simulink model "ssc_car_fuel_cell_1motor"  (R2026a)
settings: Solver=daessc  StopTime=195  FixedStep=1e-3  AbsTol=1e-3
InitFcn:
  | %Vehicle = sm_car_vehcfg_checkConfig(Vehicle);
undefined symbols (not defined in the file): Control, Driver, Init, Maneuver1, Vehicle
libraries: fl_lib x93, nesl_utility x38, GasN_lib x21, sdl_lib x10, simulink_extras x6, SimscapeFluids_lib x6, simulink x5, customMath_lib x5, slpidlib x4, ee_lib x3, autolibshared x2, sl_discontinuities x2
(part 3 of 4)

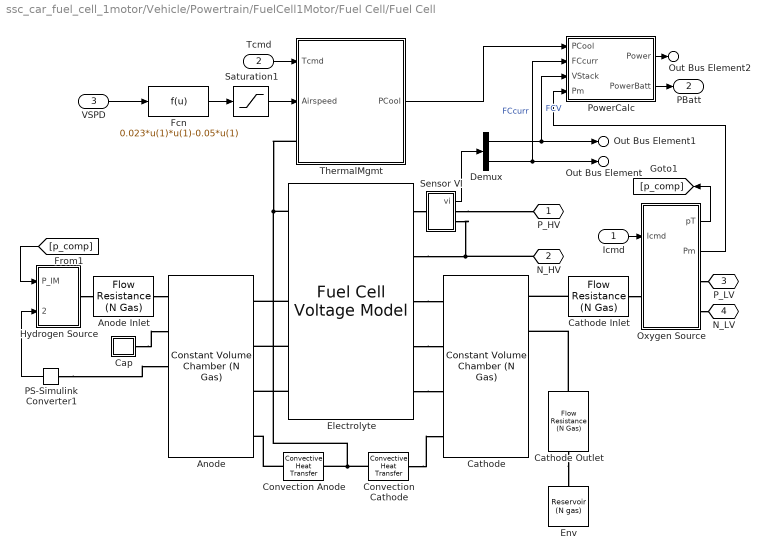
== system ssc_car_fuel_cell_1motor/Vehicle/Powertrain/FuelCell1Motor/Fuel Cell/Fuel Cell ==
  Icmd : Inport
  Tcmd : Inport  Port=2
  VSPD : Inport  Port=3
  Anode : GasN_lib/Constant Volume Chamber (N Gas)  V0=FuelCell.Anode.volume.Value m^3  p0=FuelCell.Anode.p.Value MPa  T0=FuelCell.Anode.T.Value degC  comp=GasN.composition_enum.mole  y0=FuelCell.Anode.rMoleFractions.Value'  x0=[1; 0; 0; 0]  tau_c=FuelCell.Anode.timeCondensation.Value s  is_cond=FuelCell.Anode.speciesCondensed.Value'  out_comp=GasN.composition_enum.mass  area_A=FuelCell.Anode.areaPort.Value cm^2  area_B=FuelCell.Anode.areaPort.Value cm^2  area_C=FuelCell.Anode.areaPort.Value cm^2
  Anode Inlet : GasN_lib/Flow Resistance (N Gas)  var_res=false  delta_p_nominal="FuelCell.AnodeInlet.pDropNominal.Value  MPa"  mdot_nominal=FuelCell.AnodeInlet.mdotNominal.Value kg/s  rho_nominal="FuelCell.AnodeInlet.rhoNominal.Value  kg/m^3"  laminar_fraction=FuelCell.AnodeInlet.rmdotLaminar.Value  area=FuelCell.AnodeInlet.areaPort.Value cm^2  leak_thresh=FuelCell.AnodeInlet.leakageThreshold.Value
  Cap : Subsystem
  Cathode : GasN_lib/Constant Volume Chamber (N Gas)  V0=FuelCell.Cathode.volume.Value m^3  p0=FuelCell.Cathode.p.Value MPa  T0=FuelCell.Cathode.T.Value degC  comp=GasN.composition_enum.mole  y0=FuelCell.Cathode.rMoleFractions.Value'  x0=[1; 0; 0; 0]  tau_c=FuelCell.Cathode.timeCondensation.Value s  is_cond=FuelCell.Cathode.speciesCondensed.Value'  out_comp=GasN.composition_enum.mass  area_A=FuelCell.Cathode.areaPort.Value cm^2  area_B=FuelCell.Cathode.areaPort.Value cm^2  area_C=FuelCell.Cathode.areaPort.Value cm^2
  Cathode Inlet : GasN_lib/Flow Resistance (N Gas)  var_res=false  delta_p_nominal=FuelCell.CathodeInlet.pDropNominal.Value MPa  mdot_nominal=FuelCell.CathodeInlet.mdotNominal.Value kg/s  rho_nominal="FuelCell.CathodeInlet.rhoNominal.Value  kg/m^3"  laminar_fraction=FuelCell.CathodeInlet.rmdotLaminar.Value  area=FuelCell.CathodeInlet.areaPort.Value cm^2  leak_thresh=FuelCell.CathodeInlet.leakageThreshold.Value
  Cathode Outlet : GasN_lib/Flow Resistance (N Gas)  var_res=false  delta_p_nominal=FuelCell.CathodeOutlet.pDropNominal.Value MPa  mdot_nominal=FuelCell.CathodeOutlet.mdotNominal.Value kg/s  rho_nominal=FuelCell.CathodeOutlet.rhoNominal.Value kg/m^3  laminar_fraction=FuelCell.CathodeOutlet.rmdotLaminar.Value  area=FuelCell.CathodeOutlet.areaPort.Value cm^2  leak_thresh=FuelCell.CathodeOutlet.leakageThreshold.Value
  Convection Anode : fl_lib/Thermal/Thermal Elements/Convective Heat Transfer  thermal_type=foundation.enum.constant_variable.constant  area=280*400/8 cm^2  heat_tr_coeff=10 W/(m^2 * K)  min_heat_tr_coeff=1e-3 W/(K*m^2)  T_specify=off  T_priority=None  T=0 K  T_nominal_specify=off  T_nominal_value=1  T_nominal_unit=K  Q_specify=off  Q_priority=None  Q=0 W  Q_nominal_specify=off  Q_nominal_value=1  Q_nominal_unit=W
  Convection Cathode : fl_lib/Thermal/Thermal Elements/Convective Heat Transfer  thermal_type=foundation.enum.constant_variable.constant  area=280*400/8 cm^2  heat_tr_coeff=10 W/(m^2 * K)  min_heat_tr_coeff=1e-3 W/(K*m^2)  T_specify=off  T_priority=None  T=0 K  T_nominal_specify=off  T_nominal_value=1  T_nominal_unit=K  Q_specify=off  Q_priority=None  Q=0 W  Q_nominal_specify=off  Q_nominal_value=1  Q_nominal_unit=W
  Demux : Demux  Outputs=2
  Electrolyte : gn_supplement_lib/fuel_cell/Fuel Cell Voltage Model  Ncell=FuelCell.Electrolyte.numCells.Value  Acell=FuelCell.Electrolyte.areaCell.Value cm^2  tcell=FuelCell.Electrolyte.thicknessMembrane.Value cm  io=FuelCell.Electrolyte.exchangeCurrentDensity.Value A/cm^2  iL=FuelCell.Electrolyte.maxCurrentDensity.Value A/cm^2  alpha=FuelCell.Electrolyte.transferCoefficientB.Value  rho_m=FuelCell.Electrolyte.rhoMembrane.Value kg/cm^3  M_m=FuelCell.Electrolyte.mMembrane.Value kg/mol
  Env : GasN_lib/Reservoir (N gas)  p0=FuelCell.CathodeReservoir.p.Value MPa  T0=FuelCell.CathodeReservoir.T.Value degC  constCond=true  comp=GasN.composition_enum.mole  y0=FuelCell.CathodeReservoir.rMoleFractions.Value'  x0=[1; 0; 0; 0]  area=FuelCell.CathodeReservoir.areaPort.Value cm^2
  Fcn : Fcn  Expr=0.023*u(1)*u(1)-0.05*u(1)
  Hydrogen Source : Subsystem
  Oxygen Source : Subsystem
  PS-Simulink Converter1 : nesl_utility/PS-Simulink Converter  PhysicalDomain=network_engine_domain  SubClassName=ps_output  LeftPortType=input  RightPortType=output  PseudoPeriodic=off  Frequencies=[]  VectorFormat=1-D array  Unit=Pa  AffineConversion=off
  PowerCalc : Subsystem
  Saturation1 : Saturate  UpperLimit=inf  LowerLimit=0  ZeroCross=off
  Sensor VI : Subsystem
  ThermalMgmt : Subsystem
      mask Display: image('sm_car_vehicle_power_cooling_active1loop_IMAGE.png');
  P_HV : PMIOPort  Side=Right
  N_HV : PMIOPort  Port=2  Side=Right
  P_LV : PMIOPort  Port=3  Side=Right
  N_LV : PMIOPort  Port=4  Side=Right
  Out Bus Element : Outport  PortName=m  Element=i
  Out Bus Element1 : Outport  PortName=m  Element=v
  Out Bus Element2 : Outport  PortName=m  Element=Power
  PBatt : Outport  Port=2
  wires:
  Icmd/1 -> Oxygen Source/1(Icmd)
  [p_comp] -> Hydrogen Source/1(P_IM)
  PowerCalc/1(Power) -> Out Bus Element2/1
  VSPD/1 -> Fcn/1
  Demux/2 -> PowerCalc/2(FCcurr), Out Bus Element/1  "FCcurr"
  Sensor VI/1(vi) -> Demux/1
  Fcn/1 -> Saturation1/1
  PowerCalc/2(PowerBatt) -> PBatt/1
  Tcmd/1 -> ThermalMgmt/1(Tcmd)
  Demux/1 -> PowerCalc/3(VStack), Out Bus Element1/1  "FCV"
  Oxygen Source/2(Pm) -> PowerCalc/4(Pm)
  Oxygen Source/1(pT) -> [p_comp]
  PS-Simulink Converter1/1 -> Hydrogen Source/2(P_anode)
  Saturation1/1 -> ThermalMgmt/2(Airspeed)
  ThermalMgmt/1(PCool) -> PowerCalc/1(PCool)
  connections:
  Cap/LConn1 -- Anode/RConn2
  Convection Anode/LConn1 -- Anode/LConn4
  Convection Cathode/LConn1 -- Cathode/LConn4
  Electrolyte/RConn3 -- Cathode/LConn1
  Electrolyte/RConn1 -- Sensor VI/LConn1
  Sensor VI/RConn1 -- P_HV/RConn1
  Cathode Inlet/RConn1 -- Cathode/RConn1
  Anode Inlet/RConn1 -- Anode/RConn1
  Electrolyte/LConn4 -- Anode/LConn2
  Electrolyte/RConn4 -- Cathode/LConn2
  PS-Simulink Converter1/LConn1 -- Anode/RConn3
  Oxygen Source/RConn2 -- N_LV/RConn1
  Hydrogen Source/RConn1 -- Anode Inlet/LConn1
  Electrolyte/RConn5 -- Cathode/LConn3
  Electrolyte/LConn5 -- Anode/LConn3
  Cathode Outlet/RConn1 -- Env/LConn1
  Cathode Inlet/LConn1 -- Oxygen Source/LConn1
  Oxygen Source/RConn1 -- P_LV/RConn1
  Electrolyte/LConn3 -- Anode/LConn1
  Cathode Outlet/LConn1 -- Cathode/RConn2
  Convection Anode/RConn1 -- Convection Cathode/RConn1 -- Electrolyte/LConn1 -- ThermalMgmt/LConn1
  Sensor VI/RConn2 -- Electrolyte/RConn2 -- N_HV/RConn1

== system ssc_car_fuel_cell_1motor/Vehicle/Powertrain/FuelCell1Motor/Fuel Cell/Thermal ==
  Controlled Heat Flow Rate Source : fl_lib/Thermal/Thermal Sources/Controlled Heat Flow Rate Source
  PS Gain : fl_lib/Physical Signals/Functions/PS Gain  Commented=on  gain=FuelCell.Converter.resistance.Value Ohm
  PS Math Function : fl_lib/Physical Signals/Functions/PS Math Function  Commented=on  fcn_choice=foundation.enum.math_function.square  v=1
  PS Power Function : customMath_lib/PS Power Function  resistance=FuelCell.Converter.resistance.Value Ohm
  Thermal Mass : fl_lib/Thermal/Thermal Elements/Thermal Mass  mass_type=foundation.enum.constant_variable.constant  mass=FuelCell.Converter.mThermal.Value kg  sp_heat=FuelCell.Converter.Cp.Value J/kg/K  mass_min=1e-6 kg  num_ports=foundation.enum.numPorts2.one  m_specify=off  m_priority=High  m=1 kg  m_nominal_specify=off  m_nominal_value=1  m_nominal_unit=kg  T_specify=off  T_priority=High  T=300 K  T_nominal_specify=off  T_nominal_value=1  T_nominal_unit=K  Q_specify=off  Q_priority=None  Q=0 W  Q_nominal_specify=off  Q_nominal_value=1  Q_nominal_unit=W
  Thermal Resistance : fl_lib/Thermal/Thermal Elements/Thermal Resistance  resistance=FuelCell.Converter.rConvection.Value K/W  T_specify=off  T_priority=None  T=0 K  T_nominal_specify=off  T_nominal_value=1  T_nominal_unit=K  Q_specify=off  Q_priority=None  Q=0 W  Q_nominal_specify=off  Q_nominal_value=1  Q_nominal_unit=W
  Thermal Reference2 : fl_lib/Thermal/Thermal Elements/Thermal Reference
  H : PMIOPort  Side=Right
  i : PMIOPort  Port=2  Side=Left
  connections:
  H/RConn1 -- Thermal Resistance/RConn1
  PS Power Function/LConn1 -- i/RConn1
  Thermal Reference2/LConn1 -- Controlled Heat Flow Rate Source/RConn2
  Controlled Heat Flow Rate Source/LConn1 -- Thermal Mass/LConn1 -- Thermal Resistance/LConn1
  PS Math Function/RConn1 -- PS Gain/LConn1
  PS Power Function/RConn1 -- Controlled Heat Flow Rate Source/RConn1

== system ssc_car_fuel_cell_1motor/Vehicle/Powertrain/FuelCell1Motor/Motor A1/Sensing Current ==
  Current Sensor : fl_lib/Electrical/Electrical Sensors/Current Sensor
  PS-Simulink Converter : nesl_utility/PS-Simulink Converter  PhysicalDomain=network_engine_domain  SubClassName=ps_output  LeftPortType=input  RightPortType=output  PseudoPeriodic=off  Frequencies=[]  VectorFormat=1-D array  Unit=A  AffineConversion=off
  + : PMIOPort  Side=Right
  - : PMIOPort  Port=2  Side=Left
  i : Outport
  wires:
  PS-Simulink Converter/1 -> i/1
  connections:
  Current Sensor/RConn2 -- -/RConn1
  Current Sensor/LConn1 -- +/RConn1
  PS-Simulink Converter/LConn1 -- Current Sensor/RConn1

== system ssc_car_fuel_cell_1motor/Vehicle/Powertrain/FuelCell1Motor/Motor A1/Sensing Torque ==
  PS-Simulink Converter : nesl_utility/PS-Simulink Converter  PhysicalDomain=network_engine_domain  SubClassName=ps_output  LeftPortType=input  RightPortType=output  PseudoPeriodic=off  Frequencies=[]  VectorFormat=1-D array  Unit=N*m  AffineConversion=off
  Torque Sensor : fl_lib/Mechanical/Mechanical Sensors/Ideal Torque Sensor
  C : PMIOPort  Side=Right
  R : PMIOPort  Port=2  Side=Left
  trq : Outport
  wires:
  PS-Simulink Converter/1 -> trq/1
  connections:
  Torque Sensor/LConn1 -- R/RConn1
  Torque Sensor/RConn1 -- C/RConn1
  Torque Sensor/RConn2 -- PS-Simulink Converter/LConn1

== system ssc_car_fuel_cell_1motor/Vehicle/Powertrain/FuelCell1Motor/Thermal System/Pump Control ==
  TAmb : Inport
  TMotor : Inport  Port=2
  Add : Sum  Inputs=|-+
  PID Controller : slpidlib/PID Controller  Controller=PI  Form=Parallel  TimeDomain=Continuous-time  UseExternalTs=off  SampleTime=-1  IntegratorMethod=Forward Euler  FilterMethod=Forward Euler  ControllerParametersSource=internal  P=Cooling.Control.Kp.Value  I=Cooling.Control.Ki.Value  UseKiTs=off  D=0  UseExternalDerivativeSource=off  N=100  UseFilter=on  TunerSelectOption=Transfer Function Based (PID Tuner App)  ZeroCross=off  InitialConditionSource=internal  InitialConditionForIntegrator=0  InitialConditionForFilter=0  DifferentiatorICPrevScaledInput=0  ExternalReset=none  TrackingMode=off  Kt=1  LimitOutput=on  SatLimitsSource=internal  UpperSaturationLimit=0.1  LowerSaturationLimit=0  LinearizeAsGain=on  AntiWindupMode=none  Kb=1  LimitIntegrator=off  UpperIntegratorSaturationLimit=inf  LowerIntegratorSaturationLimit=-inf  POutMin=[]  POutMax=[]  IOutMin=[]  IOutMax=[]  DOutMin=[]  DOutMax=[]  NOutMin=[]  NOutMax=[]  SumOutMin=[]  SumOutMax=[]  SaturationOutMin=[]  SaturationOutMax=[]  PParamMin=[]  PParamMax=[]  IParamMin=[]  IParamMax=[]  DParamMin=[]  DParamMax=[]  NParamMin=[]  NParamMax=[]  KbParamMin=[]  KbParamMax=[]  KtParamMin=[]  KtParamMax=[]  KbOutMin=[]  KbOutMax=[]  KtOutMin=[]  KtOutMax=[]  IntegratorOutMin=[]  IntegratorOutMax=[]  FilterOutMin=[]  FilterOutMax=[]  SumI1OutMin=[]  SumI1OutMax=[]  SumI2OutMin=[]  SumI2OutMax=[]  SumI3OutMin=[]  SumI3OutMax=[]  SumI4OutMin=[]  SumI4OutMax=[]  SumDOutMin=[]  SumDOutMax=[]  DifferentiatorOutMin=[]  DifferentiatorOutMax=[]  FilterDiffOutCoefMin=[]  FilterDiffOutCoefMax=[]  ReciprocalOutMin=[]  ReciprocalOutMax=[]  SumDenOutMin=[]  SumDenOutMax=[]  SumNumOutMin=[]  SumNumOutMax=[]  DivideOutMin=[]  DivideOutMax=[]  UdiffTsProdOutMin=[]  UdiffTsProdOutMax=[]  NTsProdOutMin=[]  NTsProdOutMax=[]  UintegralTsProdOutMin=[]  UintegralTsProdOutMax=[]  UngainTsProdOutMin=[]  UngainTsProdOutMax=[]  ClampingZeroOutDataTypeStr=Inherit: Inherit via back propagation  ClampingZeroOutMin=[]  ClampingZeroOutMax=[]  FilterDenConstantOutDataTypeStr=Inherit: Inherit via back propagation  FilterDenConstantOutMin=[]  FilterDenConstantOutMax=[]  PCopyOutDataTypeStr=Inherit: Inherit via back propagation  PCopyOutMin=[]  PCopyOutMax=[]  NCopyOutDataTypeStr=Inherit: Inherit via back propagation  NCopyOutMin=[]  NCopyOutMax=[]  IntegratorContinuousStateAttributes=''  IntegratorStateMustResolveToSignalObject=off  IntegratorRTWStateStorageClass=Auto  FilterContinuousStateAttributes=''  FilterStateMustResolveToSignalObject=off  FilterRTWStateStorageClass=Auto  ParallelPVariant=InternalParameters  IdealPVariant=Disabled  IVariant=InternalParameters  DVariant=Disabled  IntegratorVariant=Continuous  SatVariant=Enabled  AWVariant=Passthrough  PCopyVariant=Disabled  TRVariant=Disabled  FdbkBlocksVariant=Forward  IdealPFdbkVariant=Disabled  SatFdbkVariant=Disabled  DerivativeFilterVariant=Disabled  NVariant=Disabled  NCopyVariant=Disabled_SignalSpec  FilterICVariant=Disabled  IntegratorICVariant=InternalICs  ExternalResetVariant=Disabled  TRSumVariant=Passthrough  SumFdbkVariant=Disabled  SumVariant=Sum_PI  TsampFilterVariant=InternalTs  TsampNgainVariant=Passthrough  TsampIntegralVariant=Disabled_SignalSpec  ExternalSaturationOutDataTypeStr=Inherit: Same as second input  DerivativeSourceVariant=Disabled  PreIntVariant=InternalPreInt
  Transfer Fcn : TransferFcn  Denominator=[0.1 1]
  Pump_flw : Outport
  wires:
  Transfer Fcn/1 -> Pump_flw/1
  TMotor/1 -> Add/2
  TAmb/1 -> Add/1
  PID Controller/1 -> Transfer Fcn/1  "Pump_flw"
  Add/1 -> PID Controller/1

== system ssc_car_fuel_cell_1motor/Vehicle/Powertrain/FuelCell1Motor/Thermal System/Sensing T Amb ==
  PS-Simulink Converter1 : nesl_utility/PS-Simulink Converter  PhysicalDomain=network_engine_domain  SubClassName=ps_output  LeftPortType=input  RightPortType=output  PseudoPeriodic=off  Frequencies=[]  VectorFormat=1-D array  Unit=K  AffineConversion=off
  Temperature Sensor : fl_lib/Thermal/Thermal Sensors/Temperature Sensor  temperature_measure=foundation.enum.MeasurementReference.difference
  Thermal Reference : fl_lib/Thermal/Thermal Elements/Thermal Reference
  A : PMIOPort  Side=Left
  T : Outport
  wires:
  PS-Simulink Converter1/1 -> T/1
  connections:
  Temperature Sensor/RConn1 -- Thermal Reference/LConn1
  Temperature Sensor/RConn2 -- PS-Simulink Converter1/LConn1
  Temperature Sensor/LConn1 -- A/RConn1

== system ssc_car_fuel_cell_1motor/Vehicle/Powertrain/FuelCell1Motor/Thermal System/Sensing T Conv ==
  PS-Simulink Converter1 : nesl_utility/PS-Simulink Converter  PhysicalDomain=network_engine_domain  SubClassName=ps_output  LeftPortType=input  RightPortType=output  PseudoPeriodic=off  Frequencies=[]  VectorFormat=1-D array  Unit=K  AffineConversion=off
  Temperature Sensor : fl_lib/Thermal/Thermal Sensors/Temperature Sensor  temperature_measure=foundation.enum.MeasurementReference.difference
  Thermal Reference : fl_lib/Thermal/Thermal Elements/Thermal Reference
  A : PMIOPort  Side=Left
  T : Outport
  wires:
  PS-Simulink Converter1/1 -> T/1
  connections:
  Temperature Sensor/RConn1 -- Thermal Reference/LConn1
  Temperature Sensor/RConn2 -- PS-Simulink Converter1/LConn1
  Temperature Sensor/LConn1 -- A/RConn1

== system ssc_car_fuel_cell_1motor/Vehicle/Powertrain/FuelCell1Motor/Thermal System/Sensing T MotorR ==
  PS-Simulink Converter1 : nesl_utility/PS-Simulink Converter  PhysicalDomain=network_engine_domain  SubClassName=ps_output  LeftPortType=input  RightPortType=output  PseudoPeriodic=off  Frequencies=[]  VectorFormat=1-D array  Unit=K  AffineConversion=off
  Temperature Sensor : fl_lib/Thermal/Thermal Sensors/Temperature Sensor  temperature_measure=foundation.enum.MeasurementReference.difference
  Thermal Reference : fl_lib/Thermal/Thermal Elements/Thermal Reference
  A : PMIOPort  Side=Left
  T : Outport
  wires:
  PS-Simulink Converter1/1 -> T/1
  connections:
  Temperature Sensor/LConn1 -- A/RConn1
  Temperature Sensor/RConn2 -- PS-Simulink Converter1/LConn1
  Temperature Sensor/RConn1 -- Thermal Reference/LConn1

== system ssc_car_fuel_cell_1motor/Vehicle/Powertrain/FuelCell1Motor/Thermal System/Tank ==
  Absolute Reference (TL) : fl_lib/Thermal Liquid/Elements/Absolute Reference (TL)
  Cap (G) : fl_lib/Gas/Elements/Cap (G)  p_specify=off  p_priority=None  p=0.101325 MPa  p_nominal_specify=off  p_nominal_value=1  p_nominal_unit=MPa  T_specify=off  T_priority=None  T=293.15 K  T_nominal_specify=off  T_nominal_value=1  T_nominal_unit=K
  Convection HGas : fl_lib/Thermal/Thermal Elements/Convective Heat Transfer  thermal_type=foundation.enum.constant_variable.constant  area=1e-2 m^2  heat_tr_coeff=20 W/(m^2 * K)  min_heat_tr_coeff=1e-3 W/(K*m^2)  T_specify=off  T_priority=None  T=0 K  T_nominal_specify=off  T_nominal_value=1  T_nominal_unit=K  Q_specify=off  Q_priority=None  Q=0 W  Q_nominal_specify=off  Q_nominal_value=1  Q_nominal_unit=W
  Convection HLiq : fl_lib/Thermal/Thermal Elements/Convective Heat Transfer  thermal_type=foundation.enum.constant_variable.constant  area=1e-4 m^2  heat_tr_coeff=20 W/(m^2 * K)  min_heat_tr_coeff=1e-3 W/(K*m^2)  T_specify=off  T_priority=None  T=0 K  T_nominal_specify=off  T_nominal_value=1  T_nominal_unit=K  Q_specify=off  Q_priority=None  Q=0 W  Q_nominal_specify=off  Q_nominal_value=1  Q_nominal_unit=W
  Flow Resistance (G) : fl_lib/Gas/Elements/Flow Resistance (G)  delta_p_nominal=0.001 MPa  mdot_nominal=0.1 kg/s  rho_nominal=0 kg/m^3  area=0.01 m^2  laminar_fraction=1e-3
  Reservoir (G) : fl_lib/Gas/Elements/Reservoir (G)  pressure_input=false  pressure_spec=1  reservoir_pressure=0.101325 MPa  temperature_input=false  reservoir_temperature=25 degC  area_A=0.001 m^2  input_error_spec=foundation.enum.input_range_error.warn
  Sensor P T : fl_lib/Thermal Liquid/Sensors/Pressure & Temperature Sensor (TL)  reference=foundation.enum.MeasurementReference.difference  pressure=true  pressure_spec=foundation.enum.PressureMeasementSpec.Absolute  temperature=true
  Tank : SimscapeFluids_lib/Thermal Liquid/Tanks & Accumulators/Tank (G-TL)  num_inlet=2  volume_total=Cooling.Tank.volume.Value m^3  volume_spec=1  tank_area=Cooling.Tank.area.Value m^2  level_TLU=[0, 3, 5] m  volume_TLU=[0, 4, 6] m^3  inlet_areas_A1B1=Cooling.Tank.areaA1B1.Value m^2  inlet_height_A2=0.1 m  inlet_area_A2=0.01 m^2  inlet_heights_A2B2=Cooling.Tank.heightA2B2.Value m  inlet_areas_A2B2=Cooling.Tank.areaA2B2.Value m^2  inlet_heights_A2B2C2=[.1, .1, .1] m  inlet_areas_A2B2C2=[.01, .01, .01] m^2  inlet_heights_A2B2C2D2=0.1 * ones(1, 4) m  inlet_areas_A2B2C2D2=0.01 * ones(1, 4) m^2  inlet_heights_A2B2C2D2E2=0.1 * ones(1, 5) m  inlet_areas_A2B2C2D2E2=0.01 * ones(1, 5) m^2  inlet_heights_A2B2C2D2E2F2=0.1 * ones(1, 6) m  inlet_areas_A2B2C2D2E2F2=0.01 * ones(1, 6) m^2  capacity_check=0  max_liquid_capacity=Cooling.Tank.volume.Value m^3  g=9.81 m/s^2  level_specify=on  level_priority=High  level="Cooling.Tank.heightInit.Value  m"  level_nominal_specify=off  level_nominal_value=1  level_nominal_unit=m  volume_liquid_specify=off  volume_liquid_priority=None  volume_liquid=5 m^3  volume_liquid_nominal_specify=off  volume_liquid_nominal_value=1  volume_liquid_nominal_unit=m^3  mass_liquid_specify=off  mass_liquid_priority=None  mass_liquid=5e+3 kg  mass_liquid_nominal_specify=off  mass_liquid_nominal_value=1  mass_liquid_nominal_unit=kg  T_liquid_specify=on  T_liquid_priority=High  T_liquid=Cooling.Tank.TliquidInit.Value K  T_liquid_nominal_specify=off  T_liquid_nominal_value=1  T_liquid_nominal_unit=K  p_gas_specify=off  p_gas_priority=High  p_gas=0.101325 MPa  p_gas_nominal_specify=off  p_gas_nominal_value=1  p_gas_nominal_unit=MPa  T_gas_specify=on  T_gas_priority=High  T_gas=Cooling.Tank.TgasInit.Value K  T_gas_nominal_specify=off  T_gas_nominal_value=1  T_gas_nominal_unit=K  rho_gas_specify=off  rho_gas_priority=None  rho_gas=1.2 kg/m^3  rho_gas_nominal_specify=off  rho_gas_nominal_value=1  rho_gas_nominal_unit=kg/m^3
  B : PMIOPort  Side=Left
  HGas : PMIOPort  Port=2  Side=Left
  A : PMIOPort  Port=3  Side=Right
  HLiq : PMIOPort  Port=4  Side=Left
  T : PMIOPort  Port=5  Side=Right
  connections:
  Tank/RConn1 -- Convection HGas/LConn1
  Convection HLiq/RConn1 -- HLiq/RConn1
  Sensor P T/RConn3 -- T/RConn1
  Sensor P T/RConn1 -- Absolute Reference (TL)/LConn1
  B/RConn1 -- Sensor P T/LConn1 -- Tank/LConn4
  Cap (G)/LConn1 -- Tank/LConn2
  Convection HGas/RConn1 -- HGas/RConn1
  Reservoir (G)/LConn1 -- Flow Resistance (G)/LConn1
  Tank/RConn2 -- Convection HLiq/LConn1
  Tank/LConn3 -- A/RConn1
  Flow Resistance (G)/RConn1 -- Tank/LConn1

== system ssc_car_fuel_cell_1motor/Vehicle/Powertrain/FuelCell1Motor/Thermal System/Thermal Circuit Converter FC ==
  Conductive Heat Transfer : fl_lib/Thermal/Thermal Elements/Conductive Heat Transfer  thermal_type=foundation.enum.ConstantVariableTabulated.Constant  wall_geometry=foundation.enum.ConductionWallGeometry.Planar  area=Cooling.Converter.conductionArea.Value m^2  thickness=Cooling.Converter.conductionThickness.Value m  d_in=0.05 m  d_out=0.1 m  L=1 m  th_cond_min=10 W/(K*m)  th_cond=Cooling.Converter.conductivity.Value W/(m*K)  th_cond_TLU=[413, 401, 392, 383, 371, 357, 342] W/(K*m)  temp_TLU=[200, 273, 400, 600, 800, 1000, 1200] K  T_specify=off  T_priority=None  T=0 K  T_nominal_specify=off  T_nominal_value=1  T_nominal_unit=K  Q_specify=off  Q_priority=None  Q=0 W  Q_nominal_specify=off  Q_nominal_value=1  Q_nominal_unit=W
  Thermal Mass : fl_lib/Thermal/Thermal Elements/Thermal Mass  mass_type=foundation.enum.constant_variable.constant  mass=Cooling.Converter.mThermal.Value kg  sp_heat=Cooling.Converter.Cp.Value J/kg/K  mass_min=1e-6 kg  num_ports=foundation.enum.numPorts2.one  m_specify=off  m_priority=High  m=1 kg  m_nominal_specify=off  m_nominal_value=1  m_nominal_unit=kg  T_specify=off  T_priority=High  T=300 K  T_nominal_specify=off  T_nominal_value=1  T_nominal_unit=K  Q_specify=off  Q_priority=None  Q=0 W  Q_nominal_specify=off  Q_nominal_value=1  Q_nominal_unit=W
  A : PMIOPort  Side=Left
  B : PMIOPort  Port=2  Side=Right
  connections:
  Conductive Heat Transfer/LConn1 -- A/RConn1
  B/RConn1 -- Thermal Mass/LConn1 -- Conductive Heat Transfer/RConn1

== system ssc_car_fuel_cell_1motor/Vehicle/Powertrain/FuelCell1Motor/Thermal System/Thermal Circuit MotorA1 ==
  Case-Ambient Insulated : fl_lib/Thermal/Thermal Elements/Perfect Insulator  T_specify=off  T_priority=None  T=0 K  T_nominal_specify=off  T_nominal_value=1  T_nominal_unit=K
  Iron Stack-Case Conductance : fl_lib/Thermal/Thermal Elements/Conductive Heat Transfer  thermal_type=foundation.enum.ConstantVariableTabulated.Constant  wall_geometry=foundation.enum.ConductionWallGeometry.Planar  area=Cooling.MotorA1.statorArea.Value cm^2  thickness=Cooling.MotorA1.statorThickness.Value cm  d_in=0.05 m  d_out=0.1 m  L=1 m  th_cond_min=10 W/(K*m)  th_cond=Cooling.MotorA1.statorConductivity.Value W/(m*K)  th_cond_TLU=[413, 401, 392, 383, 371, 357, 342] W/(K*m)  temp_TLU=[200, 273, 400, 600, 800, 1000, 1200] K  T_specify=off  T_priority=None  T=0 K  T_nominal_specify=off  T_nominal_value=1  T_nominal_unit=K  Q_specify=off  Q_priority=None  Q=0 W  Q_nominal_specify=off  Q_nominal_value=1  Q_nominal_unit=W
  Motor Case Thermal Mass : fl_lib/Thermal/Thermal Elements/Thermal Mass  mass_type=foundation.enum.constant_variable.constant  mass=Cooling.MotorA1.statormThermal.Value kg  sp_heat="Cooling.MotorA1.statorCp.Value  J/kg/K"  mass_min=1e-6 kg  num_ports=foundation.enum.numPorts2.one  m_specify=off  m_priority=High  m=1 kg  m_nominal_specify=off  m_nominal_value=1  m_nominal_unit=kg  T_specify=off  T_priority=High  T=300 K  T_nominal_specify=off  T_nominal_value=1  T_nominal_unit=K  Q_specify=off  Q_priority=None  Q=0 W  Q_nominal_specify=off  Q_nominal_value=1  Q_nominal_unit=W
  Stator Iron Thermal Mass : fl_lib/Thermal/Thermal Elements/Thermal Mass  mass_type=foundation.enum.constant_variable.constant  mass=Cooling.MotorA1.w2smThermal.Value kg  sp_heat=Cooling.MotorA1.w2sCp.Value J/kg/K  mass_min=1e-6 kg  num_ports=foundation.enum.numPorts2.one  m_specify=off  m_priority=High  m=1 kg  m_nominal_specify=off  m_nominal_value=1  m_nominal_unit=kg  T_specify=off  T_priority=High  T=300 K  T_nominal_specify=off  T_nominal_value=1  T_nominal_unit=K  Q_specify=off  Q_priority=None  Q=0 W  Q_nominal_specify=off  Q_nominal_value=1  Q_nominal_unit=W
  Winding Conductance : fl_lib/Thermal/Thermal Elements/Conductive Heat Transfer  thermal_type=foundation.enum.ConstantVariableTabulated.Constant  wall_geometry=foundation.enum.ConductionWallGeometry.Planar  area=Cooling.MotorA1.windingArea.Value cm^2  thickness=Cooling.MotorA1.windingThickness.Value cm  d_in=0.05 m  d_out=0.1 m  L=1 m  th_cond_min=10 W/(K*m)  th_cond=Cooling.MotorA1.windingConductivity.Value W/(m*K)  th_cond_TLU=[413, 401, 392, 383, 371, 357, 342] W/(K*m)  temp_TLU=[200, 273, 400, 600, 800, 1000, 1200] K  T_specify=off  T_priority=None  T=0 K  T_nominal_specify=off  T_nominal_value=1  T_nominal_unit=K  Q_specify=off  Q_priority=None  Q=0 W  Q_nominal_specify=off  Q_nominal_value=1  Q_nominal_unit=W
  Winding Thermal Mass : fl_lib/Thermal/Thermal Elements/Thermal Mass  mass_type=foundation.enum.constant_variable.constant  mass=Cooling.MotorA1.windingmThermal.Value kg  sp_heat=Cooling.MotorA1.Cp.Value J/kg/K  mass_min=1e-6 kg  num_ports=foundation.enum.numPorts2.one  m_specify=off  m_priority=High  m=1 kg  m_nominal_specify=off  m_nominal_value=1  m_nominal_unit=kg  T_specify=off  T_priority=High  T=300 K  T_nominal_specify=off  T_nominal_value=1  T_nominal_unit=K  Q_specify=off  Q_priority=None  Q=0 W  Q_nominal_specify=off  Q_nominal_value=1  Q_nominal_unit=W
  Winding-Iron Conductance : fl_lib/Thermal/Thermal Elements/Conductive Heat Transfer  thermal_type=foundation.enum.ConstantVariableTabulated.Constant  wall_geometry=foundation.enum.ConductionWallGeometry.Planar  area=Cooling.MotorA1.w2sArea.Value cm^2  thickness=Cooling.MotorA1.w2sThickness.Value cm  d_in=0.05 m  d_out=0.1 m  L=1 m  th_cond_min=10 W/(K*m)  th_cond=Cooling.MotorA1.w2sConductivity.Value W/(m*K)  th_cond_TLU=[413, 401, 392, 383, 371, 357, 342] W/(K*m)  temp_TLU=[200, 273, 400, 600, 800, 1000, 1200] K  T_specify=off  T_priority=None  T=0 K  T_nominal_specify=off  T_nominal_value=1  T_nominal_unit=K  Q_specify=off  Q_priority=None  Q=0 W  Q_nominal_specify=off  Q_nominal_value=1  Q_nominal_unit=W
  A : PMIOPort  Side=Left
  B : PMIOPort  Port=2  Side=Right
  connections:
  Winding Conductance/LConn1 -- Winding-Iron Conductance/RConn1 -- Winding Thermal Mass/LConn1
  Motor Case Thermal Mass/LConn1 -- Iron Stack-Case Conductance/RConn1 -- Case-Ambient Insulated/LConn1
  Stator Iron Thermal Mass/LConn1 -- Iron Stack-Case Conductance/LConn1 -- Winding-Iron Conductance/LConn1 -- B/RConn1
  Winding Conductance/RConn1 -- A/RConn1

== system ssc_car_fuel_cell_1motor/Vehicle/Powertrain/FuelCell1Motor/Fuel Cell/Fuel Cell/Cap ==
  Absolute Reference (N Gas) : GasN_lib/Absolute Reference (N Gas)
  Sensor P T : GasN_lib/Pressure and Temperature Sensor (N Gas)
  A : PMIOPort  Side=Left
  connections:
  Absolute Reference (N Gas)/LConn1 -- Sensor P T/RConn3
  Sensor P T/LConn1 -- A/RConn1

== system ssc_car_fuel_cell_1motor/Vehicle/Powertrain/FuelCell1Motor/Fuel Cell/Fuel Cell/Hydrogen Source ==
  P_IM : Inport
  P_anode : Inport  Port=2
  Fcn : Fcn  Expr=(0.95*u+3000)
  Gain : Gain  Gain=1/101325
  Gain1 : Gain  Gain=1/101325
  H2Side : GasN_lib/Reservoir (N gas)  p0=FuelCell.AnodeReservoir.p.Value MPa  T0=FuelCell.AnodeReservoir.T.Value degC  constCond=true  comp=GasN.composition_enum.mole  y0=FuelCell.AnodeReservoir.rMoleFractions.Value'  x0=[1; 0; 0; 0]  area=FuelCell.AnodeReservoir.areaPort.Value cm^2
  Mass Flow Rate Source (N Gas) : GasN_lib/Mass Flow Rate Source (N Gas)  const_flow=false  flow_rate=0 kg/s  power_spec=foundation.enum.power_spec.none  area_A=FuelCell.Anode.areaPort.Value cm^2  area_B=FuelCell.Anode.areaPort.Value cm^2  mdot_A_specify=off  mdot_A_priority=None  mdot_A=0.1 kg/s  mdot_A_nominal_specify=off  mdot_A_nominal_value=1  mdot_A_nominal_unit=kg/s  mdot_B_specify=off  mdot_B_priority=None  mdot_B=0.1 kg/s  mdot_B_nominal_specify=off  mdot_B_nominal_value=1  mdot_B_nominal_unit=kg/s  phi_A_specify=off  phi_A_priority=None  phi_A=0 J/s  phi_A_nominal_specify=off  phi_A_nominal_value=1  phi_A_nominal_unit=J/s  phi_B_specify=off  phi_B_priority=None  phi_B=0 J/s  phi_B_nominal_specify=off  phi_B_nominal_value=1  phi_B_nominal_unit=J/s  mdot_A_i_specify=off  mdot_A_i_priority=None  mdot_A_i=[ 0; 0; 0; 0 ] kg/s  mdot_A_i_nominal_specify=off  mdot_A_i_nominal_value=1  mdot_A_i_nominal_unit=kg/s  mdot_B_i_specify=off  mdot_B_i_priority=None  mdot_B_i=[ 0; 0; 0; 0 ] kg/s  mdot_B_i_nominal_specify=off  mdot_B_i_nominal_value=1  mdot_B_i_nominal_unit=kg/s
  Saturation : Saturate  UpperLimit=.1  LowerLimit=0.000001  ZeroCross=off
  Simulink-PS Converter5 : nesl_utility/Simulink-PS Converter  PhysicalDomain=network_engine_domain  SubClassName=ps_input  LeftPortType=input  RightPortType=output  PseudoPeriodic=off  Frequencies=[]  NoiseDistribution=none  NoiseParameters=[]  Unit=kg/s  AffineConversion=off  FilteringAndDerivatives=provide  SimscapeFilterOrder=1  InputFilterTimeConstant=0.001  UdotUserProvided=0
  Sum2 : Sum  Inputs=|+-  InputSameDT=on  SaturateOnIntegerOverflow=on  OutDataTypeStr=Inherit: Same as first input
  Transfer Fcn : TransferFcn  Denominator=[0.001 1]
  A : PMIOPort  Side=Right
  wires:
  P_anode/1 -> Gain/1
  P_IM/1 -> Fcn/1
  Sum2/1 -> Transfer Fcn/1
  Gain/1 -> Sum2/2
  Saturation/1 -> Simulink-PS Converter5/1
  Fcn/1 -> Gain1/1
  Gain1/1 -> Sum2/1
  Transfer Fcn/1 -> Saturation/1
  connections:
  H2Side/LConn1 -- Mass Flow Rate Source (N Gas)/LConn2
  Mass Flow Rate Source (N Gas)/RConn1 -- A/RConn1
  Mass Flow Rate Source (N Gas)/LConn1 -- Simulink-PS Converter5/RConn1

== system ssc_car_fuel_cell_1motor/Vehicle/Powertrain/FuelCell1Motor/Fuel Cell/Fuel Cell/Oxygen Source ==
  Icmd : Inport
  Chiller : Subsystem
  Compressor : Subsystem
  Desired RH : Constant  Value=FuelCell.Humidifier.relativeHdes.Value
  Gain : Gain  Gain=1.1
  Humidifier : Subsystem
  Saturation : Saturate  UpperLimit=inf  LowerLimit=0  ZeroCross=off
  B : PMIOPort  Side=Left
  P_LV : PMIOPort  Port=2  Side=Right
  N_LV : PMIOPort  Port=3  Side=Right
  pT : Outport
  Pm : Outport  Port=2
  wires:
  Icmd/1 -> Gain/1
  Compressor/1(pT) -> pT/1
  Desired RH/1 -> Humidifier/1(Desired RH)
  Gain/1 -> Saturation/1
  Compressor/2(Pm) -> Pm/1
  Saturation/1 -> Compressor/1(V)
  connections:
  Compressor/RConn2 -- N_LV/RConn1
  B/RConn1 -- Humidifier/RConn1
  Compressor/RConn1 -- P_LV/RConn1
  Humidifier/LConn1 -- Chiller/RConn1
  Chiller/LConn1 -- Compressor/LConn1

== system ssc_car_fuel_cell_1motor/Vehicle/Powertrain/FuelCell1Motor/Fuel Cell/Fuel Cell/PowerCalc ==
  PCool : Inport
  FCcurr : Inport  Port=2
  VStack : Inport  Port=3
  Pm : Inport  Port=4
  Product : Product
  Subtract : Sum  Inputs=+--
  Subtract1 : Sum
  Transfer Fcn (with initial outputs) : simulink_extras/Additional Linear/Transfer Fcn (with initial outputs)  N=[1]  D="[1  1]"  Y0=.5  U0=0
  Transfer Fcn (with initial outputs)1 : simulink_extras/Additional Linear/Transfer Fcn (with initial outputs)  N=[1]  D="[.1  1]"  Y0=0  U0=0
  Transfer Fcn (with initial outputs)2 : simulink_extras/Additional Linear/Transfer Fcn (with initial outputs)  N=[1]  D="[.1  1]"  Y0=0  U0=0
  Power : Outport
  PowerBatt : Outport  Port=2
  wires:
  Product/1 -> Transfer Fcn (with initial outputs)2/1  "FCpwr"
  Transfer Fcn (with initial outputs)/1 -> Subtract/2, Subtract1/1
  Subtract1/1 -> PowerBatt/1
  Transfer Fcn (with initial outputs)1/1 -> Subtract1/2, Subtract/3
  Pm/1 -> Transfer Fcn (with initial outputs)/1
  FCcurr/1 -> Product/2
  Transfer Fcn (with initial outputs)2/1 -> Subtract/1
  VStack/1 -> Product/1
  Subtract/1 -> Power/1
  PCool/1 -> Transfer Fcn (with initial outputs)1/1

== system ssc_car_fuel_cell_1motor/Vehicle/Powertrain/FuelCell1Motor/Fuel Cell/Fuel Cell/Sensor VI ==
  Current Sensor : fl_lib/Electrical/Electrical Sensors/Current Sensor
  Mux : Mux  Inputs=2
  PS-Simulink Converter2 : nesl_utility/PS-Simulink Converter  PhysicalDomain=network_engine_domain  SubClassName=ps_output  LeftPortType=input  RightPortType=output  PseudoPeriodic=off  Frequencies=[]  VectorFormat=1-D array  Unit=1  AffineConversion=off
  PS-Simulink Converter4 : nesl_utility/PS-Simulink Converter  PhysicalDomain=network_engine_domain  SubClassName=ps_output  LeftPortType=input  RightPortType=output  PseudoPeriodic=off  Frequencies=[]  VectorFormat=1-D array  Unit=1  AffineConversion=off
  Transfer Fcn1 : TransferFcn  Denominator=[.001 1]
  Transfer Fcn5 : TransferFcn  Denominator=[.001 1]
  Voltage Sensor2 : fl_lib/Electrical/Electrical Sensors/Voltage Sensor
  + : PMIOPort  Side=Left
  - : PMIOPort  Port=2  Side=Right
  G : PMIOPort  Port=3  Side=Right
  vi : Outport
  wires:
  Mux/1 -> vi/1
  Transfer Fcn5/1 -> Mux/1  "FCV"
  Transfer Fcn1/1 -> Mux/2  "FCcurr"
  PS-Simulink Converter2/1 -> Transfer Fcn1/1
  PS-Simulink Converter4/1 -> Transfer Fcn5/1
  connections:
  Current Sensor/RConn1 -- PS-Simulink Converter2/LConn1
  Voltage Sensor2/RConn2 -- G/RConn1
  Current Sensor/RConn2 -- -/RConn1
  PS-Simulink Converter4/LConn1 -- Voltage Sensor2/RConn1
  Voltage Sensor2/LConn1 -- Current Sensor/LConn1 -- +/RConn1

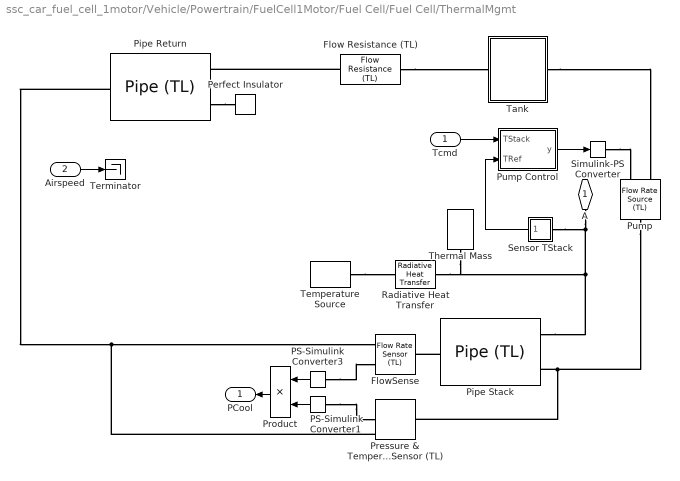
== system ssc_car_fuel_cell_1motor/Vehicle/Powertrain/FuelCell1Motor/Fuel Cell/Fuel Cell/ThermalMgmt ==
  Tcmd : Inport
  Airspeed : Inport  Port=2
  Flow Resistance (TL) : fl_lib/Thermal Liquid/Elements/Flow Resistance (TL)  delta_p_nominal=FuelCell.Thermal.Restriction.pDrop.Value MPa  mdot_nominal=FuelCell.Thermal.Restriction.mdotNominal.Value kg/s  area=FuelCell.Thermal.Restriction.areaPorts.Value m^2  laminar_fraction=FuelCell.Thermal.Restriction.rmdotLaminar.Value
  FlowSense : fl_lib/Thermal Liquid/Sensors/Flow Rate Sensor (TL)  mass_flow_measure=false  volumetric_flow_measure=true  energy_flow_measure=false
  PS-Simulink Converter1 : nesl_utility/PS-Simulink Converter  PhysicalDomain=network_engine_domain  SubClassName=ps_output  LeftPortType=input  RightPortType=output  PseudoPeriodic=off  Frequencies=[]  VectorFormat=1-D array  Unit=1  AffineConversion=off
  PS-Simulink Converter3 : nesl_utility/PS-Simulink Converter  PhysicalDomain=network_engine_domain  SubClassName=ps_output  LeftPortType=input  RightPortType=output  PseudoPeriodic=off  Frequencies=[]  VectorFormat=1-D array  Unit=1  AffineConversion=off
  Perfect Insulator : fl_lib/Thermal/Thermal Elements/Perfect Insulator  T_specify=off  T_priority=None  T=0 K  T_nominal_specify=off  T_nominal_value=1  T_nominal_unit=K
  Pipe Return : fl_lib/Thermal Liquid/Elements/Pipe (TL)  length=FuelCell.Thermal.Return.pipeLength.Value cm  area=FuelCell.Thermal.Return.pipeArea.Value cm^2  Dh=FuelCell.Thermal.Return.dHydraulic.Value cm  length_add=FuelCell.Thermal.Return.xFriction.Value m  roughness=FuelCell.Thermal.Return.roughness.Value m  Re_lam=FuelCell.Thermal.Return.laminarReynoldsMax.Value  Re_tur=FuelCell.Thermal.Return.turbulentReynoldsMin.Value  shape_factor=FuelCell.Thermal.Return.frictionDarcy.Value  Nu_lam=FuelCell.Thermal.Return.laminarNusselt.Value  dynamic_compressibility=1  inertia=0  p0=FuelCell.Thermal.Return.p.Value MPa  T0=FuelCell.Thermal.Return.T.Value degC  mdot0=0 kg/s  p_nominal=0.101325 MPa  T_nominal=293.15 K
  Pipe Stack : fl_lib/Thermal Liquid/Elements/Pipe (TL)  length=FuelCell.Thermal.FCStack.pipeLength.Value cm  area=FuelCell.Thermal.FCStack.pipeArea.Value cm^2  Dh=FuelCell.Thermal.FCStack.dHydraulic.Value cm  length_add=FuelCell.Thermal.FCStack.xFriction.Value m  roughness=FuelCell.Thermal.FCStack.roughness.Value m  Re_lam=FuelCell.Thermal.FCStack.laminarReynoldsMax.Value  Re_tur=FuelCell.Thermal.FCStack.turbulentReynoldsMin.Value  shape_factor=FuelCell.Thermal.FCStack.frictionDarcy.Value  Nu_lam=FuelCell.Thermal.FCStack.laminarNusselt.Value  dynamic_compressibility=simscape.enum.onoff.on  inertia=simscape.enum.onoff.off  p0="FuelCell.Thermal.FCStack.p.Value  MPa"  T0=FuelCell.Thermal.FCStack.T.Value degC  mdot0=0 kg/s  p_nominal=0.101325 MPa  T_nominal=293.15 K
  Pressure & Temperature Sensor (TL) : fl_lib/Thermal Liquid/Sensors/Pressure & Temperature Sensor (TL)  reference=foundation.enum.MeasurementReference.difference  pressure=true  pressure_spec=foundation.enum.PressureMeasementSpec.Absolute  temperature=true
  Product : Product
  Pump : fl_lib/Thermal Liquid/Sources/Flow Rate Source (TL)  source_type=foundation.enum.constant_controlled.controlled  flow_type=foundation.enum.mass_volumetric_flow.mass  mass_flow=0 kg/s  volumetric_flow=0 m^3/s  power_spec=foundation.enum.power_spec.isentropic  area=FuelCell.Thermal.Pump.areaPorts.Value cm^2
  Pump Control : Subsystem
  Radiative Heat Transfer : fl_lib/Thermal/Thermal Elements/Radiative Heat Transfer  area=FuelCell.Thermal.FCStack.area.Value m^2  rad_tr_coeff=FuelCell.Thermal.FCStack.kRadiation.Value W/(m^2*K^4)  T_specify=off  T_priority=None  T=0 K  T_nominal_specify=off  T_nominal_value=1  T_nominal_unit=K  Q_specify=off  Q_priority=None  Q=0 W  Q_nominal_specify=off  Q_nominal_value=1  Q_nominal_unit=W
  Sensor TStack : Subsystem
  Simulink-PS Converter : nesl_utility/Simulink-PS Converter  PhysicalDomain=network_engine_domain  SubClassName=ps_input  LeftPortType=input  RightPortType=output  PseudoPeriodic=off  Frequencies=[]  NoiseDistribution=none  NoiseParameters=[]  Unit=kg/s  AffineConversion=off  FilteringAndDerivatives=filter  SimscapeFilterOrder=1  InputFilterTimeConstant=1  UdotUserProvided=0
  Tank : Subsystem
  Temperature Source : fl_lib/Thermal/Thermal Sources/Temperature Source  temperature=FuelCell.Thermal.FCStack.Tambient.Value K
  Terminator : Terminator
  Thermal Mass : fl_lib/Thermal/Thermal Elements/Thermal Mass  mass_type=foundation.enum.constant_variable.constant  mass=FuelCell.Thermal.FCStack.mThermal.Value kg  sp_heat=FuelCell.Thermal.FCStack.Cp.Value J/kg/K  mass_min=1e-6 kg  num_ports=foundation.enum.numPorts2.one  m_specify=off  m_priority=High  m=1 kg  m_nominal_specify=off  m_nominal_value=1  m_nominal_unit=kg  T_specify=on  T_priority=High  T=353.15 K  T_nominal_specify=off  T_nominal_value=1  T_nominal_unit=K  Q_specify=off  Q_priority=None  Q=0 W  Q_nominal_specify=off  Q_nominal_value=1  Q_nominal_unit=W
  A : PMIOPort  Side=Left
  PCool : Outport
  wires:
  PS-Simulink Converter3/1 -> Product/1
  PS-Simulink Converter1/1 -> Product/2
  Sensor TStack/1(T) -> Pump Control/2(TRef)
  Pump Control/1(y) -> Simulink-PS Converter/1
  Tcmd/1 -> Pump Control/1(TStack)
  Airspeed/1 -> Terminator/1
  Product/1 -> PCool/1
  connections:
  Temperature Source/LConn1 -- Radiative Heat Transfer/RConn1
  Pump/RConn1 -- Pressure & Temperature Sensor (TL)/LConn1 -- Pipe Stack/LConn1
  Pipe Return/LConn2 -- Perfect Insulator/LConn1
  Flow Resistance (TL)/LConn1 -- Tank/LConn1
  Tank/RConn1 -- Pump/LConn1
  Flow Resistance (TL)/RConn1 -- Pipe Return/LConn1
  Pipe Return/RConn1 -- FlowSense/RConn1 -- Pressure & Temperature Sensor (TL)/RConn1
  Simulink-PS Converter/RConn1 -- Pump/LConn2
  PS-Simulink Converter3/LConn1 -- FlowSense/RConn2
  PS-Simulink Converter1/LConn1 -- Pressure & Temperature Sensor (TL)/RConn2
  Pipe Stack/RConn1 -- FlowSense/LConn1
  Sensor TStack/LConn1 -- Pipe Stack/LConn2 -- Radiative Heat Transfer/LConn1 -- Thermal Mass/LConn1 -- A/RConn1

== system ssc_car_fuel_cell_1motor/Vehicle/Powertrain/FuelCell1Motor/Fuel Cell/Fuel Cell/Oxygen Source/Chiller ==
  Heat Control : Subsystem
  Heat Flow Rate Source : fl_lib/Thermal/Thermal Sources/Controlled Heat Flow Rate Source
  Pipe : GasN_lib/Pipe (N Gas)  length=FuelCell.Chiller.xPipe.Value m  area=FuelCell.Chiller.areaPipe.Value cm^2  Dh=FuelCell.Chiller.dHydraulic.Value cm  extra_length=FuelCell.Chiller.xFriction.Value m  roughness=FuelCell.Chiller.roughness.Value m  Re_lam=FuelCell.Chiller.laminarReynoldsMax.Value  Re_tur=FuelCell.Chiller.turbulentReynoldsMin.Value  shape_factor=FuelCell.Chiller.frictionDarcy.Value  Nu_lam=FuelCell.Chiller.laminarNusselt.Value  p0=FuelCell.Chiller.p.Value MPa  T0=FuelCell.Chiller.T.Value degC  comp=GasN.composition_enum.mole  y0=FuelCell.Chiller.rMoleFractions.Value'  x0=[1; 0; 0; 0]  tau_c=FuelCell.Chiller.timeCondensation.Value s  isCond=FuelCell.Chiller.speciesCondensed.Value'
  Tdes : Constant  Value=FuelCell.Chiller.Tdesired.Value
  Thermal Reference : fl_lib/Thermal/Thermal Elements/Thermal Reference
  A : PMIOPort  Side=Left
  B : PMIOPort  Port=2  Side=Right
  wires:
  Tdes/1 -> Heat Control/1(TDes)
  connections:
  Heat Control/RConn1 -- Heat Flow Rate Source/RConn1
  A/RConn1 -- Heat Control/LConn1
  Pipe/LConn1 -- Heat Control/RConn2
  Heat Flow Rate Source/LConn1 -- Pipe/LConn2
  B/RConn1 -- Pipe/RConn1
  Thermal Reference/LConn1 -- Heat Flow Rate Source/RConn2

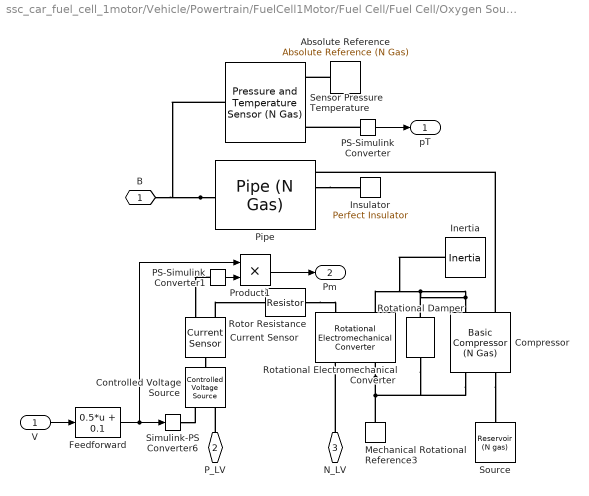
== system ssc_car_fuel_cell_1motor/Vehicle/Powertrain/FuelCell1Motor/Fuel Cell/Fuel Cell/Oxygen Source/Compressor ==
  V : Inport
  Absolute Reference : GasN_lib/Absolute Reference (N Gas)
  Compressor : GasN_lib/Basic Compressor (N Gas)  pr_des=FuelCell.Compressor.rPressure.Value  mdot_corr_des=FuelCell.Compressor.mdotDesign.Value kg/s  omega_corr_des=FuelCell.Compressor.wDesign.Value rad/s  p_ref=FuelCell.Compressor.pReference.Value MPa  T_ref=FuelCell.Compressor.TReference.Value K  RH_ref=FuelCell.Compressor.relHumidity.Value  b1=FuelCell.Compressor.kSpeedCurve.Value  b2=FuelCell.Compressor.kSpeedOffset.Value  b3=FuelCell.Compressor.kSpeedSharp.Value  eta_poly=FuelCell.Compressor.effPolytropic.Value  eta_mech=FuelCell.Compressor.effMechanical.Value  area_A=FuelCell.Compressor.areaInlet.Value cm^2  area_B=FuelCell.Compressor.areaOutlet.Value cm^2  mdot_A_specify=off  mdot_A_priority=None  mdot_A=0.1 kg/s  mdot_A_nominal_specify=off  mdot_A_nominal_value=1  mdot_A_nominal_unit=kg/s  mdot_B_specify=off  mdot_B_priority=None  mdot_B=0.1 kg/s  mdot_B_nominal_specify=off  mdot_B_nominal_value=1  mdot_B_nominal_unit=kg/s  Phi_A_specify=off  Phi_A_priority=None  Phi_A=0 J/s  Phi_A_nominal_specify=off  Phi_A_nominal_value=1  Phi_A_nominal_unit=J/s  Phi_B_specify=off  Phi_B_priority=None  Phi_B=0 J/s  Phi_B_nominal_specify=off  Phi_B_nominal_value=1  Phi_B_nominal_unit=J/s  mdot_A_i_specify=off  mdot_A_i_priority=None  mdot_A_i=[ 0; 0; 0; 0 ] kg/s  mdot_A_i_nominal_specify=off  mdot_A_i_nominal_value=1  mdot_A_i_nominal_unit=kg/s  mdot_B_i_specify=off  mdot_B_i_priority=None  mdot_B_i=[ 0; 0; 0; 0 ] kg/s  mdot_B_i_nominal_specify=off  mdot_B_i_nominal_value=1  mdot_B_i_nominal_unit=kg/s  torque_specify=off  torque_priority=None  torque=1 N*m  torque_nominal_specify=off  torque_nominal_value=1  torque_nominal_unit=N*m
  Controlled Voltage Source : fl_lib/Electrical/Electrical Sources/Controlled Voltage Source
  Current Sensor : fl_lib/Electrical/Electrical Sensors/Current Sensor
  Feedforward : Fcn  Expr=0.5*u + 0.1
  Inertia : fl_lib/Mechanical/Rotational Elements/Inertia  inertia=FuelCell.Compressor.J.Value kg*m^2  num_ports=foundation.enum.numPorts2.one  w_specify=on  w_priority=High  w=0 rad/s  w_nominal_specify=off  w_nominal_value=1  w_nominal_unit=rad/s  t_specify=off  t_priority=None  t=0 N*m  t_nominal_specify=off  t_nominal_value=1  t_nominal_unit=N*m
  Insulator : fl_lib/Thermal/Thermal Elements/Perfect Insulator  T_specify=off  T_priority=None  T=0 K  T_nominal_specify=off  T_nominal_value=1  T_nominal_unit=K
  Mechanical Rotational Reference3 : fl_lib/Mechanical/Rotational Elements/Mechanical Rotational Reference
  PS-Simulink Converter : nesl_utility/PS-Simulink Converter  PhysicalDomain=network_engine_domain  SubClassName=ps_output  LeftPortType=input  RightPortType=output  PseudoPeriodic=off  Frequencies=[]  VectorFormat=1-D array  Unit=Pa  AffineConversion=off
  PS-Simulink Converter1 : nesl_utility/PS-Simulink Converter  PhysicalDomain=network_engine_domain  SubClassName=ps_output  LeftPortType=input  RightPortType=output  PseudoPeriodic=off  Frequencies=[]  VectorFormat=1-D array  Unit=A  AffineConversion=off
  Pipe : GasN_lib/Pipe (N Gas)  length=FuelCell.CompressorPipe.xPipe.Value m  area=FuelCell.CompressorPipe.areaPipe.Value cm^2  Dh=FuelCell.CompressorPipe.dHydraulic.Value cm  extra_length=FuelCell.CompressorPipe.xFriction.Value m  roughness=FuelCell.CompressorPipe.roughness.Value m  Re_lam=FuelCell.CompressorPipe.laminarReynoldsMax.Value  Re_tur=FuelCell.CompressorPipe.turbulentReynoldsMin.Value  shape_factor=FuelCell.CompressorPipe.frictionDarcy.Value  Nu_lam=FuelCell.CompressorPipe.laminarNusselt.Value  p0=FuelCell.CompressorPipe.p.Value MPa  T0=FuelCell.CompressorPipe.T.Value degC  comp=GasN.composition_enum.mole  y0=FuelCell.CompressorPipe.rMoleFractions.Value'  x0=[1; 0; 0; 0]  tau_c=FuelCell.CompressorPipe.timeCondensation.Value s  isCond=FuelCell.CompressorPipe.speciesCondensed.Value'
  Product1 : Product
  Rotational Electromechanical Converter : fl_lib/Electrical/Electrical Elements/Rotational Electromechanical Converter  K=FuelCell.Compressor.KMotor.Value V/(rad/s)  i_specify=off  i_priority=None  i=0 A  i_nominal_specify=off  i_nominal_value=1  i_nominal_unit=A  v_specify=off  v_priority=None  v=0 V  v_nominal_specify=off  v_nominal_value=1  v_nominal_unit=V  t_specify=off  t_priority=None  t=0 N*m  t_nominal_specify=off  t_nominal_value=1  t_nominal_unit=N*m  w_specify=off  w_priority=None  w=0 rad/s  w_nominal_specify=off  w_nominal_value=1  w_nominal_unit=rad/s
  Rotational Damper : fl_lib/Mechanical/Rotational Elements/Rotational Damper  D=FuelCell.Compressor.b.Value N*m/(rad/s)  w_specify=off  w_priority=None  w=0 rad/s  w_nominal_specify=off  w_nominal_value=1  w_nominal_unit=rad/s  t_specify=off  t_priority=None  t=0 N*m  t_nominal_specify=off  t_nominal_value=1  t_nominal_unit=N*m
  Rotor Resistance : fl_lib/Electrical/Electrical Elements/Resistor  Tag=Factory Generic  R=FuelCell.Compressor.rMotor.Value Ohm  i_specify=off  i_priority=High  i=0 A  i_nominal_specify=off  i_nominal_value=1  i_nominal_unit=A  v_specify=off  v_priority=High  v=0 V  v_nominal_specify=off  v_nominal_value=1  v_nominal_unit=V
  Sensor Pressure Temperature : GasN_lib/Pressure and Temperature Sensor (N Gas)
  Simulink-PS Converter6 : nesl_utility/Simulink-PS Converter  PhysicalDomain=network_engine_domain  SubClassName=ps_input  LeftPortType=input  RightPortType=output  PseudoPeriodic=off  Frequencies=[]  NoiseDistribution=none  NoiseParameters=[]  Unit=V  AffineConversion=off  FilteringAndDerivatives=filter  SimscapeFilterOrder=1  InputFilterTimeConstant=0.01  UdotUserProvided=0
  Source : GasN_lib/Reservoir (N gas)  p0=FuelCell.CompressorSource.p.Value MPa  T0=FuelCell.CompressorSource.T.Value degC  constCond=true  comp=GasN.composition_enum.mole  y0=FuelCell.CompressorSource.rMoleFractions.Value'  x0=[1; 0; 0; 0]  area=FuelCell.CompressorSource.areaPipe.Value cm^2
  B : PMIOPort  Side=Left
  P_LV : PMIOPort  Port=2  Side=Right
  N_LV : PMIOPort  Port=3  Side=Right
  pT : Outport
  Pm : Outport  Port=2
  wires:
  Feedforward/1 -> Simulink-PS Converter6/1, Product1/1
  PS-Simulink Converter1/1 -> Product1/2
  Product1/1 -> Pm/1
  PS-Simulink Converter/1 -> pT/1
  V/1 -> Feedforward/1
  connections:
  Pipe/LConn2 -- Insulator/LConn1
  Rotor Resistance/RConn1 -- Rotational Electromechanical Converter/LConn1
  PS-Simulink Converter1/LConn1 -- Current Sensor/RConn1
  Compressor/LConn1 -- Source/LConn1
  Compressor/RConn1 -- Pipe/LConn1
  PS-Simulink Converter/LConn1 -- Sensor Pressure Temperature/RConn1
  Absolute Reference/LConn1 -- Sensor Pressure Temperature/RConn3
  Pipe/RConn1 -- Sensor Pressure Temperature/LConn1 -- B/RConn1
  Current Sensor/RConn2 -- Rotor Resistance/LConn1
  Current Sensor/LConn1 -- Controlled Voltage Source/LConn1
  Rotational Electromechanical Converter/RConn2 -- Rotational Damper/RConn1 -- Compressor/LConn2 -- Mechanical Rotational Reference3/LConn1
  N_LV/RConn1 -- Rotational Electromechanical Converter/RConn1
  P_LV/RConn1 -- Controlled Voltage Source/RConn2
  Simulink-PS Converter6/RConn1 -- Controlled Voltage Source/RConn1
  Compressor/RConn2 -- Inertia/LConn1 -- Rotational Electromechanical Converter/LConn2 -- Rotational Damper/LConn1
